simulink model "sensores_cod"  (R2021a)
settings: Solver=VariableStepAuto  StartTime=0.0  StopTime=30  RelTol=1e-3
libraries: simulink x3
settings Model: Creator=Francisco  LastModifiedBy=ronal
settings SolverCC: AlgebraicLoopSolver=TrustRegion
settings OptimizationCC: LifeSpan=inf
settings DebuggingCC: SFExecutionAtInitializationDiag=none  SFMachineParentedDataDiag=warning  ArithmeticOperatorsInVariantConditions=warning
settings SFSimCC: CustomCodeUndefinedFunction=UseInterfaceOnly
settings CodeAppCC: StateflowObjectComments=on

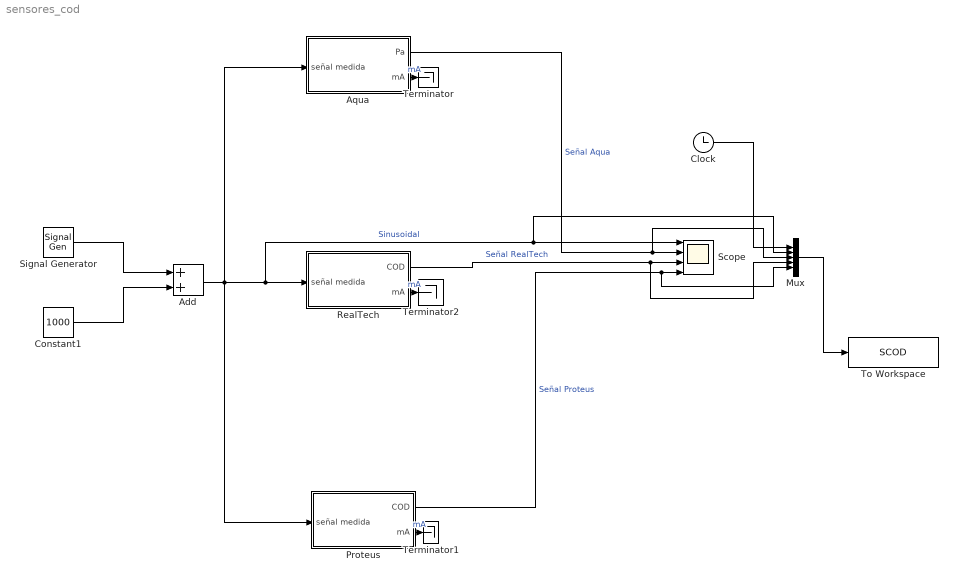
== system sensores_cod ==
  Add : Sum
  Aqua : Subsystem  mask{To=0.01, d=0, DS=2.5, Ks=0.0056, Tau=1, yo=0, Vi=1000}
      mask prompts: To "Tiempo de muestreo (s)"; d "Retardo (s)"; DS "Desviacion estandar (mg/L)"; Ks "Sensibilidad (mA/mg/L)"; Tau "Constante de tiempo (s)"; yo "Sesgo (mg/L)"; Vi "Valor inicial (mg/L)"
      mask init:
      | NP=To*DS*DS;
      mask Display: image(imread('sensor3.png'))
  Clock : Clock
  Constant1 : Constant  Value=1000
  Mux : Mux  Inputs=5
  Proteus : Subsystem  mask{To=0.01, d=0, DS=2.5, Ks=0.02667, Tau=0.33, yo=0, Vi=1000}
      mask prompts: To "Tiempo de muestreo (d)"; d "Retardo (s)"; DS "Desviacion estandar (mg/L)"; Ks "Sensibilidad (mA/mg/L)"; Tau "Constante de tiempo (d)"; yo "Sesgo (mg/L)"; Vi "Valor inicial (mg/L)"
      mask init:
      | NP=To*DS*DS;
      mask Display: image(imread('sensor1.png'))
  RealTech : Subsystem  mask{To=0.01, d=0, DS=2.5, Ks=0.0032, Tau=0.33, yo=0, Vi=1000}
      mask prompts: To "Tiempo de muestreo (d)"; d "Retardo (s)"; DS "Desviacion estandar (mg/L)"; Ks "Sensibilidad (mA/mg/L)"; Tau "Constante de tiempo (d)"; yo "Sesgo (mg/L)"; Vi "Valor inicial (mg/L)"
      mask init:
      | NP=To*DS*DS;
      mask Display: image(imread('sensor2.png'))
  Scope : Scope  NumInputPorts=4
  Signal Generator : SignalGenerator  Amplitude=100  Frequency=2/30
  Terminator : Terminator
  Terminator1 : Terminator
  Terminator2 : Terminator
  To Workspace : ToWorkspace  VariableName=SCOD  SampleTime=-1
  wires:
  Proteus/1(COD) -> Mux/5, Scope/4  "Señal Proteus"
  RealTech/1(COD) -> Mux/4, Scope/3  "Señal RealTech"
  Aqua/1(Pa) -> Mux/3, Scope/2  "Señal Aqua"
  Proteus/2(mA) -> Terminator1/1  "mA"
  RealTech/2(mA) -> Terminator2/1  "mA"
  Aqua/2(mA) -> Terminator/1  "mA"
  Signal Generator/1 -> Add/1
  Constant1/1 -> Add/2
  Add/1 -> Proteus/1(señal medida), Aqua/1(señal medida), Mux/2, Scope/1, RealTech/1(señal medida)  "Sinusoidal"
  Clock/1 -> Mux/1
  Mux/1 -> To Workspace/1

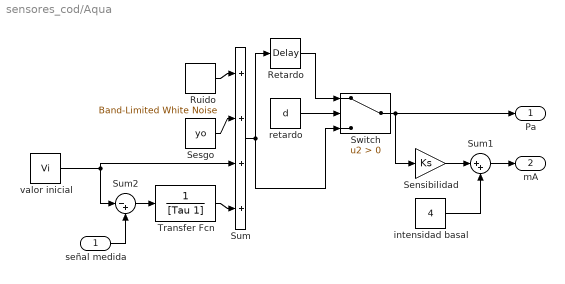
== system sensores_cod/Aqua ==
  señal medida : Inport
  Retardo : TransportDelay  DelayTime=d
  Ruido : simulink/Sources/Band-Limited White Noise  Cov=[NP]  Ts=To  seed=[23341]
  Sensibilidad : Gain  Gain=Ks
  Sesgo : Constant  Value=yo
  Sum : Sum  Inputs=|++++  SaturateOnIntegerOverflow=on
  Sum1 : Sum  Inputs=|++
  Sum2 : Sum  Inputs=|-+
  Switch : Switch  Criteria=u2 > Threshold
  Transfer Fcn : TransferFcn  Denominator=[Tau 1]
  intensidad basal : Constant  Value=4
  retardo : Constant  Value=d
  valor inicial : Constant  Value=Vi
  Pa : Outport
  mA : Outport  Port=2
  wires:
  Sensibilidad/1 -> Sum1/1
  Sum1/1 -> mA/1
  intensidad basal/1 -> Sum1/2
  retardo/1 -> Switch/2
  Sum/1 -> Retardo/1, Switch/3
  Retardo/1 -> Switch/1
  Switch/1 -> Pa/1, Sensibilidad/1
  Sesgo/1 -> Sum/2
  Ruido/1 -> Sum/1
  Transfer Fcn/1 -> Sum/4
  Sum2/1 -> Transfer Fcn/1
  señal medida/1 -> Sum2/2
  valor inicial/1 -> Sum/3, Sum2/1

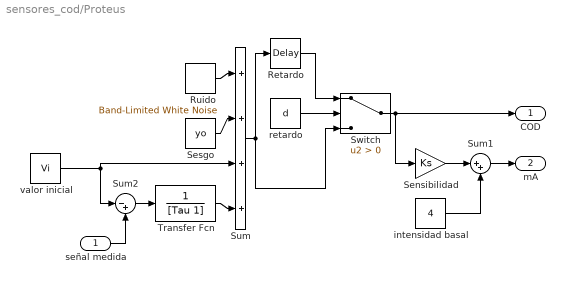
== system sensores_cod/Proteus ==
  señal medida : Inport
  Retardo : TransportDelay  DelayTime=d
  Ruido : simulink/Sources/Band-Limited White Noise  Cov=[NP]  Ts=To  seed=[23341]
  Sensibilidad : Gain  Gain=Ks
  Sesgo : Constant  Value=yo
  Sum : Sum  Inputs=|++++  SaturateOnIntegerOverflow=on
  Sum1 : Sum  Inputs=|++
  Sum2 : Sum  Inputs=|-+
  Switch : Switch  Criteria=u2 > Threshold
  Transfer Fcn : TransferFcn  Denominator=[Tau 1]
  intensidad basal : Constant  Value=4
  retardo : Constant  Value=d
  valor inicial : Constant  Value=Vi
  COD : Outport
  mA : Outport  Port=2
  wires:
  Sensibilidad/1 -> Sum1/1
  Sum1/1 -> mA/1
  intensidad basal/1 -> Sum1/2
  retardo/1 -> Switch/2
  Sum/1 -> Retardo/1, Switch/3
  Retardo/1 -> Switch/1
  Switch/1 -> COD/1, Sensibilidad/1
  Sesgo/1 -> Sum/2
  Ruido/1 -> Sum/1
  Transfer Fcn/1 -> Sum/4
  Sum2/1 -> Transfer Fcn/1
  señal medida/1 -> Sum2/2
  valor inicial/1 -> Sum/3, Sum2/1

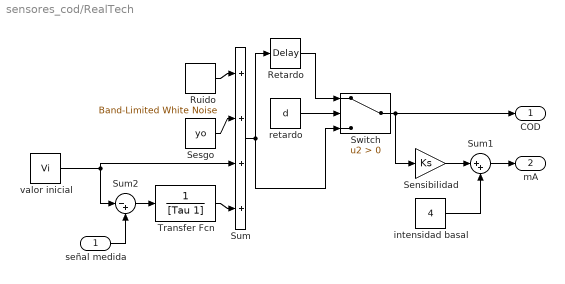
== system sensores_cod/RealTech ==
  señal medida : Inport
  Retardo : TransportDelay  DelayTime=d
  Ruido : simulink/Sources/Band-Limited White Noise  Cov=[NP]  Ts=To  seed=[23341]
  Sensibilidad : Gain  Gain=Ks
  Sesgo : Constant  Value=yo
  Sum : Sum  Inputs=|++++  SaturateOnIntegerOverflow=on
  Sum1 : Sum  Inputs=|++
  Sum2 : Sum  Inputs=|-+
  Switch : Switch  Criteria=u2 > Threshold
  Transfer Fcn : TransferFcn  Denominator=[Tau 1]
  intensidad basal : Constant  Value=4
  retardo : Constant  Value=d
  valor inicial : Constant  Value=Vi
  COD : Outport
  mA : Outport  Port=2
  wires:
  Sensibilidad/1 -> Sum1/1
  Sum1/1 -> mA/1
  intensidad basal/1 -> Sum1/2
  retardo/1 -> Switch/2
  Sum/1 -> Retardo/1, Switch/3
  Retardo/1 -> Switch/1
  Switch/1 -> COD/1, Sensibilidad/1
  Sesgo/1 -> Sum/2
  Ruido/1 -> Sum/1
  Transfer Fcn/1 -> Sum/4
  Sum2/1 -> Transfer Fcn/1
  señal medida/1 -> Sum2/2
  valor inicial/1 -> Sum/3, Sum2/1
